simulink model "agg_ut"  (Simulink 8.1)
settings: Solver=FixedStepDiscrete  StartTime=0.0  StopTime=Inf  FixedStep=0.005  RelTol=1e-3
libraries: siltestlib x3, agg x1
settings Model: Creator=xsellart  LastModifiedBy=AT015555
settings DataIOCC: SignalLoggingSaveFormat=Dataset
settings OptimizationCC: ExpressionDepthLimit=128
settings DebuggingCC: FcnCallInpInsideContextMsg=EnableAllAsError
settings GRTTargetCC: CombineOutputUpdateFcns=on  GRTInterface=off

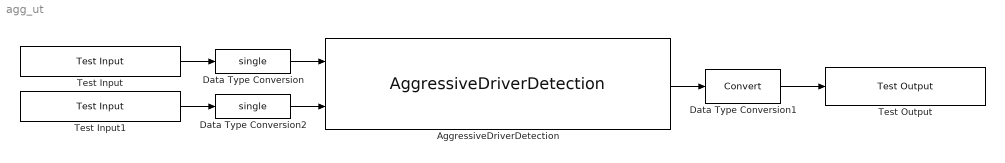
== system agg_ut ==
  AggressiveDriverDetection : agg/AggressiveDriverDetection
  Data Type Conversion : DataTypeConversion  OutDataTypeStr=single
  Data Type Conversion1 : DataTypeConversion
  Data Type Conversion2 : DataTypeConversion  OutDataTypeStr=single
  Test Input : siltestlib/Test Input  varname=VDINR_SteerSpeed_degps  sampletime=0.005
  Test Input1 : siltestlib/Test Input  varname=VDINR_HWAccelPedalPosn_pct  sampletime=0.005
  Test Output : siltestlib/Test Output  varname=VIFO_AggressiveDriverDetec_flg  sampletime=-1
  wires:
  Data Type Conversion1/1 -> Test Output/1
  Test Input/1 -> Data Type Conversion/1
  Data Type Conversion/1 -> AggressiveDriverDetection/1
  Test Input1/1 -> Data Type Conversion2/1
  Data Type Conversion2/1 -> AggressiveDriverDetection/2
  AggressiveDriverDetection/1 -> Data Type Conversion1/1
